simulink model "GunnerusDP_v1"  (R2017b)
settings: Solver=ode4  StartTime=0.0  StopTime=Tsim  FixedStep=ts  RelTol=1e-3  EnableMultiTasking=on
values from neighbouring files (symbols this model uses):
  ts = 0.01    [InitGunnerusDP.m]
undefined symbols (not defined in the file or in its folder): Control, Current, Hoerner, Par, Sim, TC_currentChange, vessel, vesselABC
libraries: marine_hydro x4, marine_gnc x3, simulink x3
(part 4 of 4)

== system GunnerusDP_v1/Environment and Vessel Dynamics/Wave definiton (from MCSim)/wave height and wave frequency/Hs and omega24/hs/If Action Subsystem1 ==
  In1 : Inport
  Action Port : ActionPort  ActionType=then
  Out1 : Outport
  wires:
  In1/1 -> Out1/1

== system GunnerusDP_v1/Environment and Vessel Dynamics/Wave definiton (from MCSim)/wave height and wave frequency/Hs and omega24/hs/If Action Subsystem2 ==
  In1 : Inport
  Action Port : ActionPort  ActionType=elseif
  Fcn : Fcn  Expr=v1-(v1-v2)/(t2-t1)*(u[1]-t1)
  Out1 : Outport
  wires:
  In1/1 -> Fcn/1
  Fcn/1 -> Out1/1

== system GunnerusDP_v1/Environment and Vessel Dynamics/Wave definiton (from MCSim)/wave height and wave frequency/Hs and omega24/hs/If Action Subsystem3 ==
  In1 : Inport
  Action Port : ActionPort  ActionType=else
  Out1 : Outport
  wires:
  In1/1 -> Out1/1

== system GunnerusDP_v1/Environment and Vessel Dynamics/Wave definiton (from MCSim)/wave height and wave frequency/Hs and omega24/omega_p/If Action Subsystem1 ==
  In1 : Inport
  Action Port : ActionPort  ActionType=then
  Out1 : Outport
  wires:
  In1/1 -> Out1/1

== system GunnerusDP_v1/Environment and Vessel Dynamics/Wave definiton (from MCSim)/wave height and wave frequency/Hs and omega24/omega_p/If Action Subsystem2 ==
  In1 : Inport
  Action Port : ActionPort  ActionType=elseif
  Fcn : Fcn  Expr=v1-(v1-v2)/(t2-t1)*(u[1]-t1)
  Out1 : Outport
  wires:
  Fcn/1 -> Out1/1
  In1/1 -> Fcn/1

== system GunnerusDP_v1/Environment and Vessel Dynamics/Wave definiton (from MCSim)/wave height and wave frequency/Hs and omega24/omega_p/If Action Subsystem3 ==
  In1 : Inport
  Action Port : ActionPort  ActionType=else
  Out1 : Outport
  wires:
  In1/1 -> Out1/1

== system GunnerusDP_v1/Environment and Vessel Dynamics/Wave definiton (from MCSim)/wave height and wave frequency/Hs and omega3/hs/If Action Subsystem1 ==
  In1 : Inport
  Action Port : ActionPort  ActionType=then
  Out1 : Outport
  wires:
  In1/1 -> Out1/1

== system GunnerusDP_v1/Environment and Vessel Dynamics/Wave definiton (from MCSim)/wave height and wave frequency/Hs and omega3/hs/If Action Subsystem2 ==
  In1 : Inport
  Action Port : ActionPort  ActionType=elseif
  Fcn : Fcn  Expr=v1-(v1-v2)/(t2-t1)*(u[1]-t1)
  Out1 : Outport
  wires:
  In1/1 -> Fcn/1
  Fcn/1 -> Out1/1

== system GunnerusDP_v1/Environment and Vessel Dynamics/Wave definiton (from MCSim)/wave height and wave frequency/Hs and omega3/hs/If Action Subsystem3 ==
  In1 : Inport
  Action Port : ActionPort  ActionType=else
  Out1 : Outport
  wires:
  In1/1 -> Out1/1

== system GunnerusDP_v1/Environment and Vessel Dynamics/Wave definiton (from MCSim)/wave height and wave frequency/Hs and omega3/omega_p/If Action Subsystem1 ==
  In1 : Inport
  Action Port : ActionPort  ActionType=then
  Out1 : Outport
  wires:
  In1/1 -> Out1/1

== system GunnerusDP_v1/Environment and Vessel Dynamics/Wave definiton (from MCSim)/wave height and wave frequency/Hs and omega3/omega_p/If Action Subsystem2 ==
  In1 : Inport
  Action Port : ActionPort  ActionType=elseif
  Fcn : Fcn  Expr=v1-(v1-v2)/(t2-t1)*(u[1]-t1)
  Out1 : Outport
  wires:
  Fcn/1 -> Out1/1
  In1/1 -> Fcn/1

== system GunnerusDP_v1/Environment and Vessel Dynamics/Wave definiton (from MCSim)/wave height and wave frequency/Hs and omega3/omega_p/If Action Subsystem3 ==
  In1 : Inport
  Action Port : ActionPort  ActionType=else
  Out1 : Outport
  wires:
  In1/1 -> Out1/1

== system GunnerusDP_v1/Environment and Vessel Dynamics/Wave definiton (from MCSim)/wave height and wave frequency/Hs and omega4/hs/If Action Subsystem1 ==
  In1 : Inport
  Action Port : ActionPort  ActionType=then
  Out1 : Outport
  wires:
  In1/1 -> Out1/1

== system GunnerusDP_v1/Environment and Vessel Dynamics/Wave definiton (from MCSim)/wave height and wave frequency/Hs and omega4/hs/If Action Subsystem2 ==
  In1 : Inport
  Action Port : ActionPort  ActionType=elseif
  Fcn : Fcn  Expr=v1-(v1-v2)/(t2-t1)*(u[1]-t1)
  Out1 : Outport
  wires:
  Fcn/1 -> Out1/1
  In1/1 -> Fcn/1

== system GunnerusDP_v1/Environment and Vessel Dynamics/Wave definiton (from MCSim)/wave height and wave frequency/Hs and omega4/hs/If Action Subsystem3 ==
  In1 : Inport
  Action Port : ActionPort  ActionType=else
  Out1 : Outport
  wires:
  In1/1 -> Out1/1

== system GunnerusDP_v1/Environment and Vessel Dynamics/Wave definiton (from MCSim)/wave height and wave frequency/Hs and omega4/omega_p/If Action Subsystem1 ==
  In1 : Inport
  Action Port : ActionPort  ActionType=then
  Out1 : Outport
  wires:
  In1/1 -> Out1/1

== system GunnerusDP_v1/Environment and Vessel Dynamics/Wave definiton (from MCSim)/wave height and wave frequency/Hs and omega4/omega_p/If Action Subsystem2 ==
  In1 : Inport
  Action Port : ActionPort  ActionType=elseif
  Fcn : Fcn  Expr=v1-(v1-v2)/(t2-t1)*(u[1]-t1)
  Out1 : Outport
  wires:
  In1/1 -> Fcn/1
  Fcn/1 -> Out1/1

== system GunnerusDP_v1/Environment and Vessel Dynamics/Wave definiton (from MCSim)/wave height and wave frequency/Hs and omega4/omega_p/If Action Subsystem3 ==
  In1 : Inport
  Action Port : ActionPort  ActionType=else
  Out1 : Outport
  wires:
  In1/1 -> Out1/1

== system GunnerusDP_v1/Environment and Vessel Dynamics/Wave definiton (from MCSim)/wave height and wave frequency/Hs and omega5/hs/If Action Subsystem1 ==
  In1 : Inport
  Action Port : ActionPort  ActionType=then
  Out1 : Outport
  wires:
  In1/1 -> Out1/1

== system GunnerusDP_v1/Environment and Vessel Dynamics/Wave definiton (from MCSim)/wave height and wave frequency/Hs and omega5/hs/If Action Subsystem2 ==
  In1 : Inport
  Action Port : ActionPort  ActionType=elseif
  Fcn : Fcn  Expr=v1-(v1-v2)/(t2-t1)*(u[1]-t1)
  Out1 : Outport
  wires:
  In1/1 -> Fcn/1
  Fcn/1 -> Out1/1

== system GunnerusDP_v1/Environment and Vessel Dynamics/Wave definiton (from MCSim)/wave height and wave frequency/Hs and omega5/hs/If Action Subsystem3 ==
  In1 : Inport
  Action Port : ActionPort  ActionType=else
  Out1 : Outport
  wires:
  In1/1 -> Out1/1

== system GunnerusDP_v1/Environment and Vessel Dynamics/Wave definiton (from MCSim)/wave height and wave frequency/Hs and omega5/omega_p/If Action Subsystem1 ==
  In1 : Inport
  Action Port : ActionPort  ActionType=then
  Out1 : Outport
  wires:
  In1/1 -> Out1/1

== system GunnerusDP_v1/Environment and Vessel Dynamics/Wave definiton (from MCSim)/wave height and wave frequency/Hs and omega5/omega_p/If Action Subsystem2 ==
  In1 : Inport
  Action Port : ActionPort  ActionType=elseif
  Fcn : Fcn  Expr=v1-(v1-v2)/(t2-t1)*(u[1]-t1)
  Out1 : Outport
  wires:
  Fcn/1 -> Out1/1
  In1/1 -> Fcn/1

== system GunnerusDP_v1/Environment and Vessel Dynamics/Wave definiton (from MCSim)/wave height and wave frequency/Hs and omega5/omega_p/If Action Subsystem3 ==
  In1 : Inport
  Action Port : ActionPort  ActionType=else
  Out1 : Outport
  wires:
  In1/1 -> Out1/1

== system GunnerusDP_v1/Environment and Vessel Dynamics/Wave definiton (from MCSim)/wave height and wave frequency/Hs and omega6/hs/If Action Subsystem1 ==
  In1 : Inport
  Action Port : ActionPort  ActionType=then
  Out1 : Outport
  wires:
  In1/1 -> Out1/1

== system GunnerusDP_v1/Environment and Vessel Dynamics/Wave definiton (from MCSim)/wave height and wave frequency/Hs and omega6/hs/If Action Subsystem2 ==
  In1 : Inport
  Action Port : ActionPort  ActionType=elseif
  Fcn : Fcn  Expr=v1-(v1-v2)/(t2-t1)*(u[1]-t1)
  Out1 : Outport
  wires:
  Fcn/1 -> Out1/1
  In1/1 -> Fcn/1

== system GunnerusDP_v1/Environment and Vessel Dynamics/Wave definiton (from MCSim)/wave height and wave frequency/Hs and omega6/hs/If Action Subsystem3 ==
  In1 : Inport
  Action Port : ActionPort  ActionType=else
  Out1 : Outport
  wires:
  In1/1 -> Out1/1

== system GunnerusDP_v1/Environment and Vessel Dynamics/Wave definiton (from MCSim)/wave height and wave frequency/Hs and omega6/omega_p/If Action Subsystem1 ==
  In1 : Inport
  Action Port : ActionPort  ActionType=then
  Out1 : Outport
  wires:
  In1/1 -> Out1/1

== system GunnerusDP_v1/Environment and Vessel Dynamics/Wave definiton (from MCSim)/wave height and wave frequency/Hs and omega6/omega_p/If Action Subsystem2 ==
  In1 : Inport
  Action Port : ActionPort  ActionType=elseif
  Fcn : Fcn  Expr=v1-(v1-v2)/(t2-t1)*(u[1]-t1)
  Out1 : Outport
  wires:
  In1/1 -> Fcn/1
  Fcn/1 -> Out1/1

== system GunnerusDP_v1/Environment and Vessel Dynamics/Wave definiton (from MCSim)/wave height and wave frequency/Hs and omega6/omega_p/If Action Subsystem3 ==
  In1 : Inport
  Action Port : ActionPort  ActionType=else
  Out1 : Outport
  wires:
  In1/1 -> Out1/1

== system GunnerusDP_v1/Environment and Vessel Dynamics/Wave definiton (from MCSim)/wave height and wave frequency/Hs and omega7/hs/If Action Subsystem1 ==
  In1 : Inport
  Action Port : ActionPort  ActionType=then
  Out1 : Outport
  wires:
  In1/1 -> Out1/1

== system GunnerusDP_v1/Environment and Vessel Dynamics/Wave definiton (from MCSim)/wave height and wave frequency/Hs and omega7/hs/If Action Subsystem2 ==
  In1 : Inport
  Action Port : ActionPort  ActionType=elseif
  Fcn : Fcn  Expr=v1-(v1-v2)/(t2-t1)*(u[1]-t1)
  Out1 : Outport
  wires:
  In1/1 -> Fcn/1
  Fcn/1 -> Out1/1

== system GunnerusDP_v1/Environment and Vessel Dynamics/Wave definiton (from MCSim)/wave height and wave frequency/Hs and omega7/hs/If Action Subsystem3 ==
  In1 : Inport
  Action Port : ActionPort  ActionType=else
  Out1 : Outport
  wires:
  In1/1 -> Out1/1

== system GunnerusDP_v1/Environment and Vessel Dynamics/Wave definiton (from MCSim)/wave height and wave frequency/Hs and omega7/omega_p/If Action Subsystem1 ==
  In1 : Inport
  Action Port : ActionPort  ActionType=then
  Out1 : Outport
  wires:
  In1/1 -> Out1/1

== system GunnerusDP_v1/Environment and Vessel Dynamics/Wave definiton (from MCSim)/wave height and wave frequency/Hs and omega7/omega_p/If Action Subsystem2 ==
  In1 : Inport
  Action Port : ActionPort  ActionType=elseif
  Fcn : Fcn  Expr=v1-(v1-v2)/(t2-t1)*(u[1]-t1)
  Out1 : Outport
  wires:
  Fcn/1 -> Out1/1
  In1/1 -> Fcn/1

== system GunnerusDP_v1/Environment and Vessel Dynamics/Wave definiton (from MCSim)/wave height and wave frequency/Hs and omega7/omega_p/If Action Subsystem3 ==
  In1 : Inport
  Action Port : ActionPort  ActionType=else
  Out1 : Outport
  wires:
  In1/1 -> Out1/1

== system GunnerusDP_v1/Environment and Vessel Dynamics/Wave definiton (from MCSim)/wave height and wave frequency/Hs and omega8/hs/If Action Subsystem1 ==
  In1 : Inport
  Action Port : ActionPort  ActionType=then
  Out1 : Outport
  wires:
  In1/1 -> Out1/1

== system GunnerusDP_v1/Environment and Vessel Dynamics/Wave definiton (from MCSim)/wave height and wave frequency/Hs and omega8/hs/If Action Subsystem2 ==
  In1 : Inport
  Action Port : ActionPort  ActionType=elseif
  Fcn : Fcn  Expr=v1-(v1-v2)/(t2-t1)*(u[1]-t1)
  Out1 : Outport
  wires:
  Fcn/1 -> Out1/1
  In1/1 -> Fcn/1

== system GunnerusDP_v1/Environment and Vessel Dynamics/Wave definiton (from MCSim)/wave height and wave frequency/Hs and omega8/hs/If Action Subsystem3 ==
  In1 : Inport
  Action Port : ActionPort  ActionType=else
  Out1 : Outport
  wires:
  In1/1 -> Out1/1

== system GunnerusDP_v1/Environment and Vessel Dynamics/Wave definiton (from MCSim)/wave height and wave frequency/Hs and omega8/omega_p/If Action Subsystem1 ==
  In1 : Inport
  Action Port : ActionPort  ActionType=then
  Out1 : Outport
  wires:
  In1/1 -> Out1/1

== system GunnerusDP_v1/Environment and Vessel Dynamics/Wave definiton (from MCSim)/wave height and wave frequency/Hs and omega8/omega_p/If Action Subsystem2 ==
  In1 : Inport
  Action Port : ActionPort  ActionType=elseif
  Fcn : Fcn  Expr=v1-(v1-v2)/(t2-t1)*(u[1]-t1)
  Out1 : Outport
  wires:
  In1/1 -> Fcn/1
  Fcn/1 -> Out1/1

== system GunnerusDP_v1/Environment and Vessel Dynamics/Wave definiton (from MCSim)/wave height and wave frequency/Hs and omega8/omega_p/If Action Subsystem3 ==
  In1 : Inport
  Action Port : ActionPort  ActionType=else
  Out1 : Outport
  wires:
  In1/1 -> Out1/1

== system GunnerusDP_v1/Environment and Vessel Dynamics/Wave definiton (from MCSim)/wave height and wave frequency/Hs and omega9/hs/If Action Subsystem1 ==
  In1 : Inport
  Action Port : ActionPort  ActionType=then
  Out1 : Outport
  wires:
  In1/1 -> Out1/1

== system GunnerusDP_v1/Environment and Vessel Dynamics/Wave definiton (from MCSim)/wave height and wave frequency/Hs and omega9/hs/If Action Subsystem2 ==
  In1 : Inport
  Action Port : ActionPort  ActionType=elseif
  Fcn : Fcn  Expr=v1-(v1-v2)/(t2-t1)*(u[1]-t1)
  Out1 : Outport
  wires:
  In1/1 -> Fcn/1
  Fcn/1 -> Out1/1

== system GunnerusDP_v1/Environment and Vessel Dynamics/Wave definiton (from MCSim)/wave height and wave frequency/Hs and omega9/hs/If Action Subsystem3 ==
  In1 : Inport
  Action Port : ActionPort  ActionType=else
  Out1 : Outport
  wires:
  In1/1 -> Out1/1

== system GunnerusDP_v1/Environment and Vessel Dynamics/Wave definiton (from MCSim)/wave height and wave frequency/Hs and omega9/omega_p/If Action Subsystem1 ==
  In1 : Inport
  Action Port : ActionPort  ActionType=then
  Out1 : Outport
  wires:
  In1/1 -> Out1/1

== system GunnerusDP_v1/Environment and Vessel Dynamics/Wave definiton (from MCSim)/wave height and wave frequency/Hs and omega9/omega_p/If Action Subsystem2 ==
  In1 : Inport
  Action Port : ActionPort  ActionType=elseif
  Fcn : Fcn  Expr=v1-(v1-v2)/(t2-t1)*(u[1]-t1)
  Out1 : Outport
  wires:
  Fcn/1 -> Out1/1
  In1/1 -> Fcn/1

== system GunnerusDP_v1/Environment and Vessel Dynamics/Wave definiton (from MCSim)/wave height and wave frequency/Hs and omega9/omega_p/If Action Subsystem3 ==
  In1 : Inport
  Action Port : ActionPort  ActionType=else
  Out1 : Outport
  wires:
  In1/1 -> Out1/1
